simulink subsystem "vmc_single_foot"  (R2022b)
settings: Solver=VariableStepAuto  StartTime=0.0  StopTime=10.0  RelTol=1e-3
model mask{P=30, D=-0.02, dir=-1, dir2=1}
  mask prompts: P "关节pd控制器比例系数P"; D "关节pd控制器微分系数D"; dir "腿部左右方向dir(左：1，右：-1）"; dir2 "腿部前后方向dir2(前：1，后：-1）"
undefined symbols (not defined in the file or in its folder): L, l1, l2, l3, W, X, Y, Z
libraries: nesl_utility x9, sm_lib x7, Contact_Forces_Lib x1
settings Model: Creator=Administrator  LastModifiedBy=LiAn

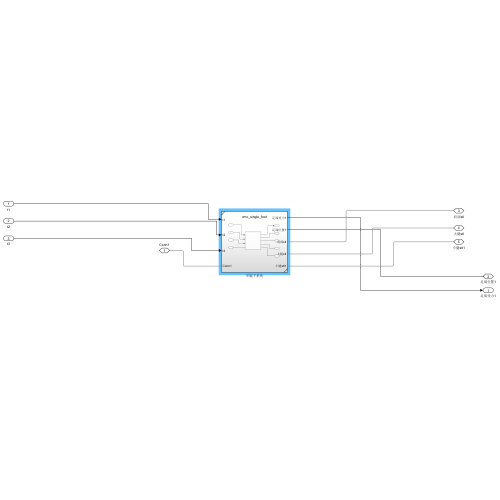
[thumbnail: Simulink's stored preview of the top-level diagram]
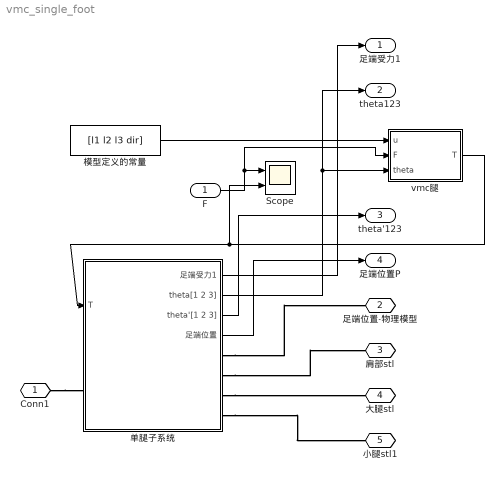
== system vmc_single_foot ==
  "F " : Inport
  Scope : Scope  NumInputPorts=2
  vmc腿 : MATLAB Function  TreatAsAtomicUnit=on
  单腿子系统 : Subsystem
  模型定义的常量 : Constant  Value=[l1 l2 l3 dir]
  Conn1 : PMIOPort  Side=Left
  足端位置-物理模型 : PMIOPort  Port=2  Side=Right
  肩部stl : PMIOPort  Port=3  Side=Right
  大腿stl : PMIOPort  Port=4  Side=Right
  小腿stl1 : PMIOPort  Port=5  Side=Right
  足端受力1 : Outport
  theta123 : Outport  Port=2
  theta'123 : Outport  Port=3
  足端位置P : Outport  Port=4
  wires:
  模型定义的常量/1 -> vmc腿/1(u)
  "F "/1 -> Scope/1, vmc腿/2(F)
  单腿子系统/1(足端受力1) -> 足端受力1/1
  单腿子系统/2(theta[1 2 3]) -> vmc腿/3(theta), theta123/1
  单腿子系统/3(theta'[1 2 3]) -> theta'123/1
  单腿子系统/4(足端位置) -> 足端位置P/1
  vmc腿/1(T) -> 单腿子系统/1(T), Scope/2
  connections:
  Conn1/RConn1 -- 单腿子系统/LConn1
  单腿子系统/RConn1 -- 足端位置-物理模型/RConn1
  单腿子系统/RConn2 -- 肩部stl/RConn1
  单腿子系统/RConn3 -- 大腿stl/RConn1
  单腿子系统/RConn4 -- 小腿stl1/RConn1

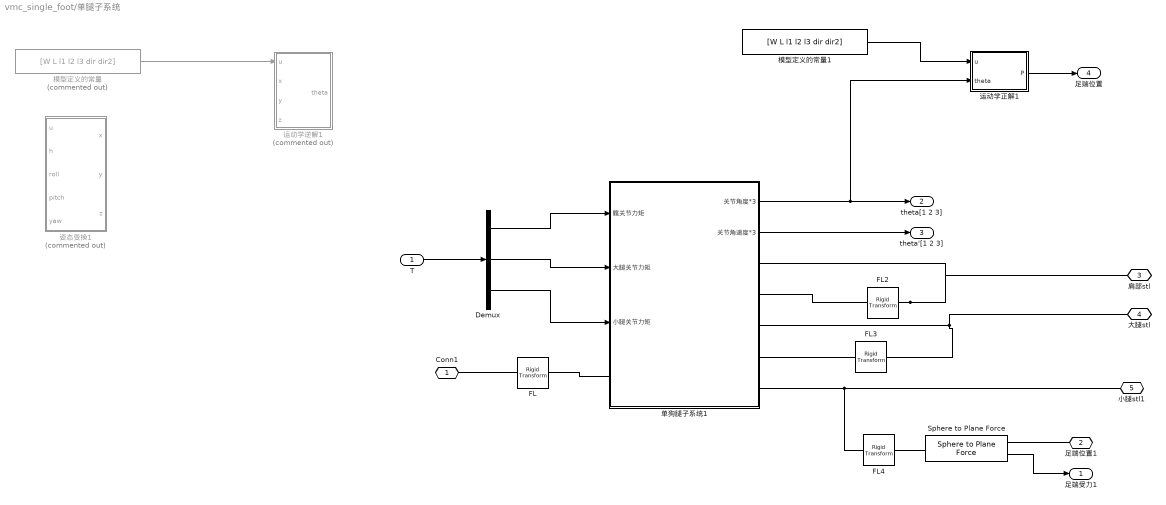
== system vmc_single_foot/单腿子系统 ==
  T : Inport
  Demux : Demux  Outputs=3
  FL : sm_lib/Frames and Transforms/Rigid Transform  TranslationMethod=Cartesian  TranslationStandardOffset=0  TranslationLengthUnit=m  TranslationStandardAxis=+Z  TranslationCartesianOffset=[dir2*L/2 dir*W/2 0]  TranslationROffset=0  TranslationROffsetUnits=m  TranslationZOffset=0  TranslationZOffsetUnits=m  TranslationThetaOffset=0  TranslationThetaOffsetUnits=deg  RotationMethod=StandardAxis  RotationAngleUnits=rad  RotationStandardAxis=+Y  RotationAngle=pi/2  RotationArbitraryAxis=[0 0 1]  FollAlignAxisA=+X  BaseAlignAxisA=+Y  FollAlignAxisB=+Y  BaseAlignAxisB=+Z  RotationSequenceAxes=FollowerAxes  RotationSequence=XYX  RotationSequenceAngles=[0 0 0]  RotationSequenceAnglesUnits=deg  RotationMatrix=[1 0 0; 0 1 0; 0 0 1]  Quaternion=[1 0 0 0]
  FL2 : sm_lib/Frames and Transforms/Rigid Transform  TranslationMethod=Cartesian  TranslationStandardOffset=0  TranslationLengthUnit=m  TranslationStandardAxis=+Z  TranslationCartesianOffset=[0 dir*l1 0]  TranslationROffset=0  TranslationROffsetUnits=m  TranslationZOffset=0  TranslationZOffsetUnits=m  TranslationThetaOffset=0  TranslationThetaOffsetUnits=deg  RotationMethod=StandardAxis  RotationAngleUnits=rad  RotationStandardAxis=-X  RotationAngle=pi/2  RotationArbitraryAxis=[0 0 1]  FollAlignAxisA=+X  BaseAlignAxisA=+Y  FollAlignAxisB=+Y  BaseAlignAxisB=+Z  RotationSequenceAxes=FollowerAxes  RotationSequence=XYX  RotationSequenceAngles=[0 0 0]  RotationSequenceAnglesUnits=deg  RotationMatrix=[1 0 0; 0 1 0; 0 0 1]  Quaternion=[1 0 0 0]
  FL3 : sm_lib/Frames and Transforms/Rigid Transform  TranslationMethod=Cartesian  TranslationStandardOffset=0  TranslationLengthUnit=m  TranslationStandardAxis=+Z  TranslationCartesianOffset=[l2 0 0]  TranslationROffset=0  TranslationROffsetUnits=m  TranslationZOffset=0  TranslationZOffsetUnits=m  TranslationThetaOffset=0  TranslationThetaOffsetUnits=deg  RotationMethod=None  RotationAngleUnits=rad  RotationStandardAxis=-X  RotationAngle=pi/2  RotationArbitraryAxis=[0 0 1]  FollAlignAxisA=+X  BaseAlignAxisA=+Y  FollAlignAxisB=+Y  BaseAlignAxisB=+Z  RotationSequenceAxes=FollowerAxes  RotationSequence=XYX  RotationSequenceAngles=[0 0 0]  RotationSequenceAnglesUnits=deg  RotationMatrix=[1 0 0; 0 1 0; 0 0 1]  Quaternion=[1 0 0 0]
  FL4 : sm_lib/Frames and Transforms/Rigid Transform  TranslationMethod=Cartesian  TranslationStandardOffset=0  TranslationLengthUnit=m  TranslationStandardAxis=+Z  TranslationCartesianOffset=[l3 0 0]  TranslationROffset=0  TranslationROffsetUnits=m  TranslationZOffset=0  TranslationZOffsetUnits=m  TranslationThetaOffset=0  TranslationThetaOffsetUnits=deg  RotationMethod=None  RotationAngleUnits=rad  RotationStandardAxis=-X  RotationAngle=pi/2  RotationArbitraryAxis=[0 0 1]  FollAlignAxisA=+X  BaseAlignAxisA=+Y  FollAlignAxisB=+Y  BaseAlignAxisB=+Z  RotationSequenceAxes=FollowerAxes  RotationSequence=XYX  RotationSequenceAngles=[0 0 0]  RotationSequenceAnglesUnits=deg  RotationMatrix=[1 0 0; 0 1 0; 0 0 1]  Quaternion=[1 0 0 0]
  Sphere to Plane Force : Contact_Forces_Lib/3D/Sphere to Plane Force  sphere_rad=0.023  plane_lenx=floor_x  plane_leny=floor_y  plane_depth=floor_h  force_law=Linear  k_contact=stiff  b_contact=damping  pen_full_damp_F=1e-4  pen_exponent=1  custom_param_1=1  custom_param_2=1  friction_law=Stick-Slip Continuous  mu_kinetic=friction_v  mu_static=friction_p  v_thr=0.001  vis_on=on  vis_opc_en=0  vis_len_plaBz=0.005  vis_clr=[1 0 0]  vis_opc=0.7
  单狗腿子系统1 : Subsystem
  姿态变换1 : MATLAB Function  Commented=on  TreatAsAtomicUnit=on
  模型定义的常量 : Constant  Commented=on  Value=[W L l1 l2 l3 dir dir2]
  模型定义的常量1 : Constant  Value=[W L l1 l2 l3 dir dir2]
  运动学正解1 : MATLAB Function  TreatAsAtomicUnit=on
  运动学逆解1 : MATLAB Function  Commented=on  TreatAsAtomicUnit=on
  Conn1 : PMIOPort  Side=Left
  足端位置1 : PMIOPort  Port=2  Side=Right
  肩部stl : PMIOPort  Port=3  Side=Right
  大腿stl : PMIOPort  Port=4  Side=Right
  小腿stl1 : PMIOPort  Port=5  Side=Right
  足端受力1 : Outport
  theta[1 2 3] : Outport  Port=2
  theta'[1 2 3] : Outport  Port=3
  足端位置 : Outport  Port=4
  wires:
  运动学正解1/1(P) -> 足端位置/1
  模型定义的常量1/1 -> 运动学正解1/1(u)
  Demux/3 -> 单狗腿子系统1/3(小腿关节力矩)
  Demux/1 -> 单狗腿子系统1/1(髋关节力矩)
  Demux/2 -> 单狗腿子系统1/2(大腿关节力矩)
  T/1 -> Demux/1
  单狗腿子系统1/2(关节角速度*3) -> theta'[1 2 3]/1
  单狗腿子系统1/1(关节角度*3) -> theta[1 2 3]/1, 运动学正解1/2(theta)
  Sphere to Plane Force/1 -> 足端受力1/1
  模型定义的常量/1 -> 运动学逆解1/1(u)
  connections:
  Conn1/RConn1 -- FL/LConn1
  FL4/RConn1 -- Sphere to Plane Force/LConn1
  单狗腿子系统1/RConn3 -- FL3/LConn1 -- 大腿stl/RConn1
  FL2/LConn1 -- 单狗腿子系统1/RConn1 -- 肩部stl/RConn1
  单狗腿子系统1/RConn2 -- FL2/RConn1
  足端位置1/RConn1 -- Sphere to Plane Force/RConn1
  FL4/LConn1 -- 单狗腿子系统1/RConn5 -- 小腿stl1/RConn1
  单狗腿子系统1/LConn1 -- FL/RConn1
  单狗腿子系统1/RConn4 -- FL3/RConn1

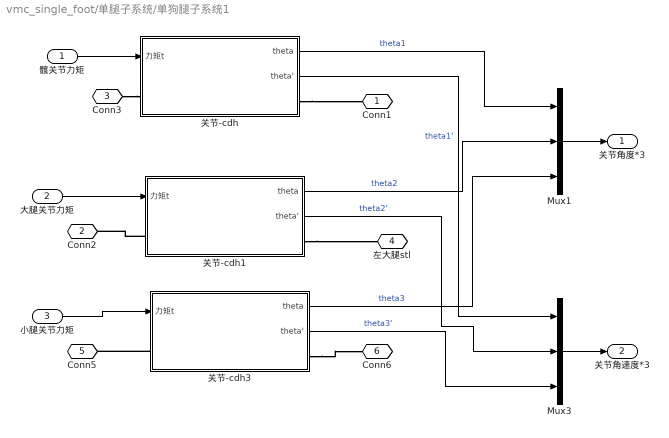
== system vmc_single_foot/单腿子系统/单狗腿子系统1 ==
  髋关节力矩 : Inport
  大腿关节力矩 : Inport  Port=2
  小腿关节力矩 : Inport  Port=3
  Mux1 : Mux  Inputs=3
  Mux3 : Mux  Inputs=3
  关节-cdh : Subsystem
  关节-cdh1 : Subsystem
  关节-cdh3 : Subsystem
  Conn1 : PMIOPort  Side=Right
  Conn2 : PMIOPort  Port=2  Side=Right
  Conn3 : PMIOPort  Port=3  Side=Left
  "左大腿stl " : PMIOPort  Port=4  Side=Right
  Conn5 : PMIOPort  Port=5  Side=Right
  Conn6 : PMIOPort  Port=6  Side=Right
  关节角度*3 : Outport
  关节角速度*3 : Outport  Port=2
  wires:
  Mux1/1 -> 关节角度*3/1
  髋关节力矩/1 -> 关节-cdh/1(力矩t)
  关节-cdh/1(theta) -> Mux1/1  "theta1"
  关节-cdh1/1(theta) -> Mux1/2  "theta2"
  关节-cdh/2(theta') -> Mux3/1  "theta1‘"
  大腿关节力矩/1 -> 关节-cdh1/1(力矩t)
  关节-cdh3/2(theta') -> Mux3/3  "theta3‘"
  Mux3/1 -> 关节角速度*3/1
  小腿关节力矩/1 -> 关节-cdh3/1(力矩t)
  关节-cdh3/1(theta) -> Mux1/3  "theta3"
  关节-cdh1/2(theta') -> Mux3/2  "theta2’"
  connections:
  关节-cdh3/RConn1 -- Conn6/RConn1
  关节-cdh1/RConn1 -- "左大腿stl "/RConn1
  关节-cdh/RConn1 -- Conn1/RConn1
  Conn3/RConn1 -- 关节-cdh/LConn1
  关节-cdh3/LConn1 -- Conn5/RConn1
  关节-cdh1/LConn1 -- Conn2/RConn1

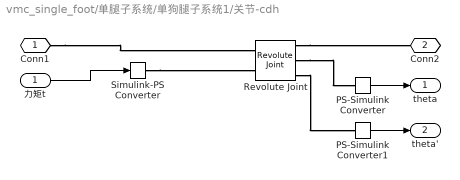
== system vmc_single_foot/单腿子系统/单狗腿子系统1/关节-cdh ==
  力矩t : Inport
  PS-Simulink Converter : nesl_utility/PS-Simulink Converter  PhysicalDomain=network_engine_domain  SubClassName=ps_output  LeftPortType=input  RightPortType=output  PseudoPeriodic=off  Frequencies=[]  VectorFormat=inherit  Unit=inherit  AffineConversion=off
  PS-Simulink Converter1 : nesl_utility/PS-Simulink Converter  PhysicalDomain=network_engine_domain  SubClassName=ps_output  LeftPortType=input  RightPortType=output  PseudoPeriodic=off  Frequencies=[]  VectorFormat=inherit  Unit=inherit  AffineConversion=off
  Revolute Joint : sm_lib/Joints/Revolute Joint  JointMode=Normal  SenseConstraintForce=off  SenseConstraintForceX=off  SenseConstraintForceY=off  SenseConstraintForceZ=off  SenseConstraintTorque=off  SenseConstraintTorqueX=off  SenseConstraintTorqueY=off  SenseConstraintTorqueZ=off  SenseTotalForce=off  SenseTotalForceX=off  SenseTotalForceY=off  SenseTotalForceZ=off  SenseTotalTorque=off  SenseTotalTorqueX=off  SenseTotalTorqueY=off  SenseTotalTorqueZ=off  CompositeWrenchDir=FollowerOnBase  CompositeWrenchFrame=BaseFrame  EquilibriumPosition=0  EquilibriumPositionUnits=deg  SpringStiffness=0  SpringStiffnessUnits=N*m/deg  DampingCoefficient=0.02  DampingCoefficientUnits=N*m/(deg/s)  TorqueActuationMode=InputTorque  MotionActuationMode=ComputedMotion  SensePosition=on  SenseVelocity=on  SenseAcceleration=off  SenseTorqueForce=off  SenseLowerLimitTorqueForce=off  SenseUpperLimitTorqueForce=off  LowerLimitSpecify=on  LowerLimitBound=-3.14  LowerLimitBoundUnits=rad  LowerLimitStiffness=1e4  LowerLimitStiffnessUnits=N*m/deg  LowerLimitDamping=10  LowerLimitDampingUnits=N*m/(deg/s)  LowerLimitTransitionRegionWidth=0.1  LowerLimitTransitionRegionWidthUnits=deg  UpperLimitSpecify=on  UpperLimitBound=3.14  UpperLimitBoundUnits=rad  UpperLimitStiffness=1e4  UpperLimitStiffnessUnits=N*m/deg  UpperLimitDamping=10  UpperLimitDampingUnits=N*m/(deg/s)  UpperLimitTransitionRegionWidth=0.1  UpperLimitTransitionRegionWidthUnits=deg  PositionTargetSpecify=off  PositionTargetPriority=High  PositionTargetValue=0  PositionTargetValueUnits=deg  VelocityTargetSpecify=off  VelocityTargetPriority=High  VelocityTargetValue=0  VelocityTargetValueUnits=deg/s
  Simulink-PS Converter : nesl_utility/Simulink-PS Converter  PhysicalDomain=network_engine_domain  SubClassName=ps_input  LeftPortType=input  RightPortType=output  PseudoPeriodic=off  Frequencies=[]  NoiseDistribution=none  NoiseParameters=[]  Unit=1  AffineConversion=off  FilteringAndDerivatives=provide  SimscapeFilterOrder=1  InputFilterTimeConstant=0.001  UdotUserProvided=0
  Conn1 : PMIOPort  Side=Left
  Conn2 : PMIOPort  Port=2  Side=Right
  theta : Outport
  theta' : Outport  Port=2
  wires:
  PS-Simulink Converter1/1 -> theta'/1
  PS-Simulink Converter/1 -> theta/1
  力矩t/1 -> Simulink-PS Converter/1
  connections:
  Revolute Joint/RConn3 -- PS-Simulink Converter1/LConn1
  Revolute Joint/RConn2 -- PS-Simulink Converter/LConn1
  Simulink-PS Converter/RConn1 -- Revolute Joint/LConn2
  Conn1/RConn1 -- Revolute Joint/LConn1
  Revolute Joint/RConn1 -- Conn2/RConn1

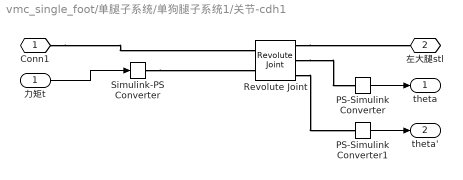
== system vmc_single_foot/单腿子系统/单狗腿子系统1/关节-cdh1 ==
  力矩t : Inport
  PS-Simulink Converter : nesl_utility/PS-Simulink Converter  PhysicalDomain=network_engine_domain  SubClassName=ps_output  LeftPortType=input  RightPortType=output  PseudoPeriodic=off  Frequencies=[]  VectorFormat=inherit  Unit=inherit  AffineConversion=off
  PS-Simulink Converter1 : nesl_utility/PS-Simulink Converter  PhysicalDomain=network_engine_domain  SubClassName=ps_output  LeftPortType=input  RightPortType=output  PseudoPeriodic=off  Frequencies=[]  VectorFormat=inherit  Unit=inherit  AffineConversion=off
  Revolute Joint : sm_lib/Joints/Revolute Joint  JointMode=Normal  SenseConstraintForce=off  SenseConstraintForceX=off  SenseConstraintForceY=off  SenseConstraintForceZ=off  SenseConstraintTorque=off  SenseConstraintTorqueX=off  SenseConstraintTorqueY=off  SenseConstraintTorqueZ=off  SenseTotalForce=off  SenseTotalForceX=off  SenseTotalForceY=off  SenseTotalForceZ=off  SenseTotalTorque=off  SenseTotalTorqueX=off  SenseTotalTorqueY=off  SenseTotalTorqueZ=off  CompositeWrenchDir=FollowerOnBase  CompositeWrenchFrame=BaseFrame  EquilibriumPosition=0  EquilibriumPositionUnits=deg  SpringStiffness=0  SpringStiffnessUnits=N*m/deg  DampingCoefficient=0.02  DampingCoefficientUnits=N*m/(deg/s)  TorqueActuationMode=InputTorque  MotionActuationMode=ComputedMotion  SensePosition=on  SenseVelocity=on  SenseAcceleration=off  SenseTorqueForce=off  SenseLowerLimitTorqueForce=off  SenseUpperLimitTorqueForce=off  LowerLimitSpecify=on  LowerLimitBound=-3.14  LowerLimitBoundUnits=rad  LowerLimitStiffness=1e4  LowerLimitStiffnessUnits=N*m/deg  LowerLimitDamping=10  LowerLimitDampingUnits=N*m/(deg/s)  LowerLimitTransitionRegionWidth=0.1  LowerLimitTransitionRegionWidthUnits=deg  UpperLimitSpecify=on  UpperLimitBound=3.14  UpperLimitBoundUnits=rad  UpperLimitStiffness=1e4  UpperLimitStiffnessUnits=N*m/deg  UpperLimitDamping=10  UpperLimitDampingUnits=N*m/(deg/s)  UpperLimitTransitionRegionWidth=0.1  UpperLimitTransitionRegionWidthUnits=deg  PositionTargetSpecify=on  PositionTargetPriority=High  PositionTargetValue=45  PositionTargetValueUnits=deg  VelocityTargetSpecify=off  VelocityTargetPriority=High  VelocityTargetValue=0  VelocityTargetValueUnits=deg/s
  Simulink-PS Converter : nesl_utility/Simulink-PS Converter  PhysicalDomain=network_engine_domain  SubClassName=ps_input  LeftPortType=input  RightPortType=output  PseudoPeriodic=off  Frequencies=[]  NoiseDistribution=none  NoiseParameters=[]  Unit=1  AffineConversion=off  FilteringAndDerivatives=provide  SimscapeFilterOrder=1  InputFilterTimeConstant=0.001  UdotUserProvided=0
  Conn1 : PMIOPort  Side=Left
  "左大腿stl " : PMIOPort  Port=2  Side=Right
  theta : Outport
  theta' : Outport  Port=2
  wires:
  力矩t/1 -> Simulink-PS Converter/1
  PS-Simulink Converter1/1 -> theta'/1
  PS-Simulink Converter/1 -> theta/1
  connections:
  Conn1/RConn1 -- Revolute Joint/LConn1
  Revolute Joint/RConn3 -- PS-Simulink Converter1/LConn1
  Revolute Joint/RConn1 -- "左大腿stl "/RConn1
  Revolute Joint/RConn2 -- PS-Simulink Converter/LConn1
  Simulink-PS Converter/RConn1 -- Revolute Joint/LConn2

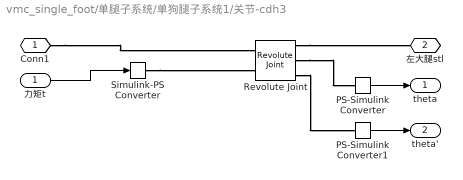
== system vmc_single_foot/单腿子系统/单狗腿子系统1/关节-cdh3 ==
  力矩t : Inport
  PS-Simulink Converter : nesl_utility/PS-Simulink Converter  PhysicalDomain=network_engine_domain  SubClassName=ps_output  LeftPortType=input  RightPortType=output  PseudoPeriodic=off  Frequencies=[]  VectorFormat=inherit  Unit=inherit  AffineConversion=off
  PS-Simulink Converter1 : nesl_utility/PS-Simulink Converter  PhysicalDomain=network_engine_domain  SubClassName=ps_output  LeftPortType=input  RightPortType=output  PseudoPeriodic=off  Frequencies=[]  VectorFormat=inherit  Unit=inherit  AffineConversion=off
  Revolute Joint : sm_lib/Joints/Revolute Joint  JointMode=Normal  SenseConstraintForce=off  SenseConstraintForceX=off  SenseConstraintForceY=off  SenseConstraintForceZ=off  SenseConstraintTorque=off  SenseConstraintTorqueX=off  SenseConstraintTorqueY=off  SenseConstraintTorqueZ=off  SenseTotalForce=off  SenseTotalForceX=off  SenseTotalForceY=off  SenseTotalForceZ=off  SenseTotalTorque=off  SenseTotalTorqueX=off  SenseTotalTorqueY=off  SenseTotalTorqueZ=off  CompositeWrenchDir=FollowerOnBase  CompositeWrenchFrame=BaseFrame  EquilibriumPosition=0  EquilibriumPositionUnits=deg  SpringStiffness=0  SpringStiffnessUnits=N*m/deg  DampingCoefficient=0.02  DampingCoefficientUnits=N*m/(deg/s)  TorqueActuationMode=InputTorque  MotionActuationMode=ComputedMotion  SensePosition=on  SenseVelocity=on  SenseAcceleration=off  SenseTorqueForce=off  SenseLowerLimitTorqueForce=off  SenseUpperLimitTorqueForce=off  LowerLimitSpecify=on  LowerLimitBound=-3.14  LowerLimitBoundUnits=rad  LowerLimitStiffness=1e4  LowerLimitStiffnessUnits=N*m/deg  LowerLimitDamping=10  LowerLimitDampingUnits=N*m/(deg/s)  LowerLimitTransitionRegionWidth=0.1  LowerLimitTransitionRegionWidthUnits=deg  UpperLimitSpecify=on  UpperLimitBound=3.14  UpperLimitBoundUnits=rad  UpperLimitStiffness=1e4  UpperLimitStiffnessUnits=N*m/deg  UpperLimitDamping=10  UpperLimitDampingUnits=N*m/(deg/s)  UpperLimitTransitionRegionWidth=0.1  UpperLimitTransitionRegionWidthUnits=deg  PositionTargetSpecify=on  PositionTargetPriority=High  PositionTargetValue=-75  PositionTargetValueUnits=deg  VelocityTargetSpecify=off  VelocityTargetPriority=High  VelocityTargetValue=0  VelocityTargetValueUnits=deg/s
  Simulink-PS Converter : nesl_utility/Simulink-PS Converter  PhysicalDomain=network_engine_domain  SubClassName=ps_input  LeftPortType=input  RightPortType=output  PseudoPeriodic=off  Frequencies=[]  NoiseDistribution=none  NoiseParameters=[]  Unit=1  AffineConversion=off  FilteringAndDerivatives=provide  SimscapeFilterOrder=1  InputFilterTimeConstant=0.001  UdotUserProvided=0
  Conn1 : PMIOPort  Side=Left
  "左大腿stl " : PMIOPort  Port=2  Side=Right
  theta : Outport
  theta' : Outport  Port=2
  wires:
  PS-Simulink Converter/1 -> theta/1
  PS-Simulink Converter1/1 -> theta'/1
  力矩t/1 -> Simulink-PS Converter/1
  connections:
  Simulink-PS Converter/RConn1 -- Revolute Joint/LConn2
  Revolute Joint/RConn2 -- PS-Simulink Converter/LConn1
  Revolute Joint/RConn1 -- "左大腿stl "/RConn1
  Revolute Joint/RConn3 -- PS-Simulink Converter1/LConn1
  Conn1/RConn1 -- Revolute Joint/LConn1

== matlab function vmc_single_foot/vmc腿 ==
  data: u input; T output; F input; theta input
function T = fcn(u,F,theta)


l1 = u(1);
l2 = u(2);
l3 = u(3);
dir = u(4);
l1 = dir*u(1);
theta1 = theta(1);
theta2 = theta(2);
theta3 = theta(3);
J_transpose = [0, l1*sin(theta1) - l3*(cos(theta1)*sin(theta2)*sin(theta3) - cos(theta1)*cos(theta2)*cos(theta3)) + l2*cos(theta1)*cos(theta2), l2*cos(theta2)*sin(theta1) - l1*cos(theta1) - l3*(sin(theta1)*sin(theta2)*sin(theta3) - cos(theta2)*cos(theta3)*sin(theta1)); - l3*(cos(theta2)*cos(theta3) - sin(theta2)*sin(theta3)) - l2*cos(theta2), - l3*(cos(theta2)*sin(theta1)*sin(theta3) + cos(theta3)*sin(theta1)*sin(theta2)) - l2*sin(theta1)*sin(theta2), l3*(cos(theta1)*cos(theta2)*sin(theta3) + cos(theta1)*cos(theta3)*sin(theta2)) + l2*cos(theta1)*sin(theta2); -l3*(cos(theta2)*cos(theta3) - sin(theta2)*sin(theta3)), -l3*(cos(theta2)*sin(theta1)*sin(theta3) + cos(theta3)*sin(theta1)*sin(theta2)), l3*(cos(theta1)*cos(theta2)*sin(theta3) + cos(theta1)*cos(theta3)*sin(theta2))];

T = J_transpose*F;

end

== matlab function vmc_single_foot/单腿子系统/姿态变换1 ==
  data: x output; u input; y output; z output; h input; roll input; pitch input; yaw input
function [x, y, z] = fcn(u,h,roll,pitch,yaw)

L = u(1);
W = u(2);
l1 = u(3);
l2 = u(4);
l3 = u(5);
dir = u(6);
dir2 = u(7);

M =[
[                               cos(pitch)*cos(yaw),                               -cos(pitch)*sin(yaw),            sin(pitch)];
[cos(roll)*sin(yaw) + cos(yaw)*sin(pitch)*sin(roll), cos(roll)*cos(yaw) - sin(pitch)*sin(roll)*sin(yaw), -cos(pitch)*sin(roll)];
[sin(roll)*sin(yaw) - cos(roll)*cos(yaw)*sin(pitch), cos(yaw)*sin(roll) + cos(roll)*sin(pitch)*sin(yaw),  cos(pitch)*cos(roll)]
];

OD = [dir2*L/2;dir*(W/2+l1);0];
OO = [0;0;h];
OA = M*[dir2*L/2;dir*(W/2);0];

AD = -OO-OA+OD;
x = AD(1,1);
y = AD(2,1);
z = AD(3,1);
end

== matlab function vmc_single_foot/单腿子系统/运动学正解1 ==
  data: u input; P output; theta input
function P = fcn(u,theta)
 

L = u(1);
W = u(2);
l1 = u(3);
l2 = u(4);
l3 = u(5);
dir = u(6);
dir2 = u(7);

%%dir:左1右-1
%%dir2:前1后-1
 
B  =    [[ 0    0   1  0];
         [ 0    1   0  0];
         [ -1   0   0  0];
         [ 0    0   0  1]];


T_01 = [[cos(theta(1))  -sin(theta(1))  0  0];
        [sin(theta(1))   cos(theta(1))  0  0];
        [          0             0  1  0];
        [          0             0  0  1]];

%T_12经历了沿y轴的平移，且额外多了个绕x轴旋转-pi/2，最后是绕z轴旋转theta,合成之后如下：
T_12 = [[cos(theta(2))  -sin(theta(2))  0  0];
        [ 0             0               0  dir*l1];
        [-sin(theta(2))  -cos(theta(2))  1  0];
        [          0             0  0  1]];

T_23 = [[cos(theta(3))  -sin(theta(3))  0  l2];
        [sin(theta(3))   cos(theta(3))  0  0];
        [          0             0  1  0];
        [          0             0  0  1]];

T_34 = [[          1             0  0  l3];
        [          0             1  0  0];
        [          0             0  1  0];
        [          0             0  0  1]];
 

%% 正向运动学矩阵
% T = B1*T_01*T_12*T_23*T_34;%% 可以通过替换参数直接求取结果
T = B*T_01*T_12*T_23*T_34;               %% 可以通过替换参数直接求取结果
R = T(1:3,1:3);
P = T(1:3,4);

== matlab function vmc_single_foot/单腿子系统/运动学逆解1 ==
  data: u input; theta output; x input; y input; z input
%单腿运动学逆解
function theta= fcn(u,x,y,z)
%P里面包含了x,y,z

L = u(1);
W = u(2);
l1 = u(3);
l2 = u(4);
l3 = u(5);
dir = u(6);
dir2 = u(7);

 
 
%肩部旋转量求解
dyz=sqrt(y^2+z^2);
lyz=sqrt(dyz^2-l1^2);
gamma_yz=-atan(y/z);
gamma_h_offset=dir*atan(l1/lyz);   
gamma=gamma_yz-gamma_h_offset;
 
%小腿旋转量求解
lxzp=sqrt(lyz^2+x^2);
n=(lxzp^2-l3^2-l2^2)/(2*l2);
beta=-acos(n/l3);
%大腿旋转量求解
alfa_xzp=-atan(x/lyz);
alfa_off=acos((l2+n)/lxzp);
alfa=(alfa_xzp+alfa_off);
 
theta = [ gamma  alfa beta ];
 
end
